simulink model "top"  (R2023a)
settings: Solver=VariableStepAuto  StartTime=0.0  StopTime=10.0  RelTol=1e-3
libraries: simulink x3
settings Model: DataDictionary=topDictionary2.sldd  Creator=Francesco  LastModifiedBy=Francesco

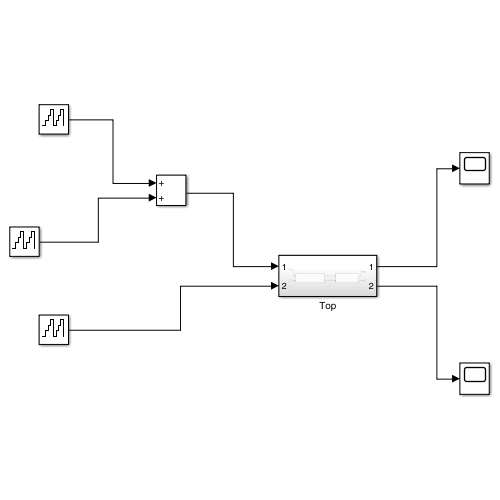
[thumbnail: Simulink's stored preview of the top-level diagram]
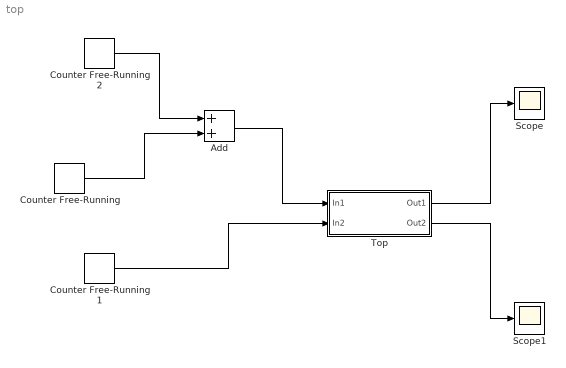
== system top ==
  Add : Sum
  Counter Free-Running : simulink/Sources/Counter Free-Running  NumBits=16  tsamp=-1
  Counter Free-Running1 : simulink/Sources/Counter Free-Running  NumBits=16  tsamp=-1
  Counter Free-Running2 : simulink/Sources/Counter Free-Running  NumBits=16  tsamp=-1
  Scope : Scope
  Scope1 : Scope
  Top : Subsystem
  wires:
  Counter Free-Running1/1 -> Top/2(In2)
  Top/1(Out1) -> Scope/1
  Top/2(Out2) -> Scope1/1
  Counter Free-Running2/1 -> Add/1
  Counter Free-Running/1 -> Add/2
  Add/1 -> Top/1(In1)

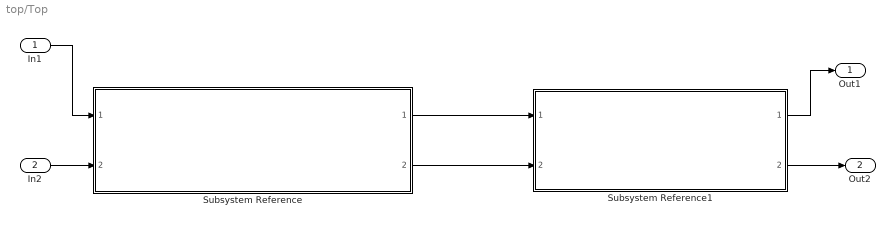
== system top/Top ==
  In1 : Inport
  In2 : Inport  Port=2
  Subsystem Reference : Subsystem  ReferencedSubsystem=modA_subsys
  Subsystem Reference1 : Subsystem  ReferencedSubsystem=modB_sys
  Out1 : Outport
  Out2 : Outport  Port=2
  wires:
  Subsystem Reference/1 -> Subsystem Reference1/1
  Subsystem Reference/2 -> Subsystem Reference1/2
  In1/1 -> Subsystem Reference/1
  In2/1 -> Subsystem Reference/2
  Subsystem Reference1/1 -> Out1/1
  Subsystem Reference1/2 -> Out2/1
